simulink model "PatientSimulator_MIMO_toTrim"  (R2022a)
settings: Solver=VariableStepAuto  StartTime=0.0  StopTime=10.0  RelTol=1e-3
undefined symbols (not defined in the file or in its folder): patient, propofol, RASS, remifentanil
libraries: cstblocks x2
settings Model: Creator=user  LastModifiedBy=user

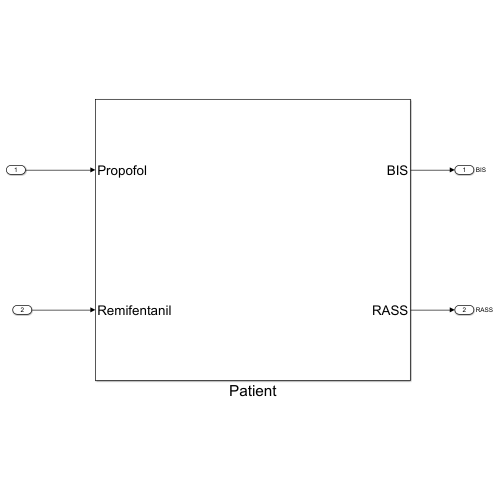
[thumbnail: Simulink's stored preview of the top-level diagram]
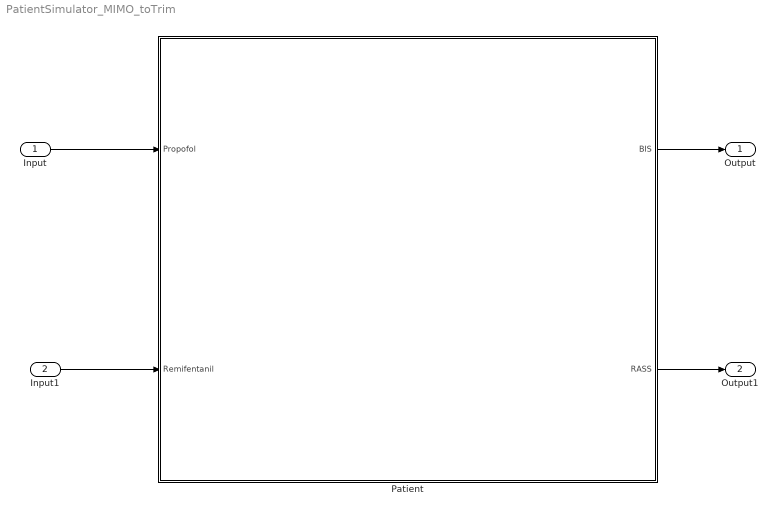
== system PatientSimulator_MIMO_toTrim ==
  Input : Inport
  Input1 : Inport  Port=2
  Patient : Subsystem
  Output : Outport  SignalName=BIS
  Output1 : Outport  Port=2  SignalName=RASS
  wires:
  Input/1 -> Patient/1(Propofol)
  Input1/1 -> Patient/2(Remifentanil)
  Patient/1(BIS) -> Output/1
  Patient/2(RASS) -> Output1/1

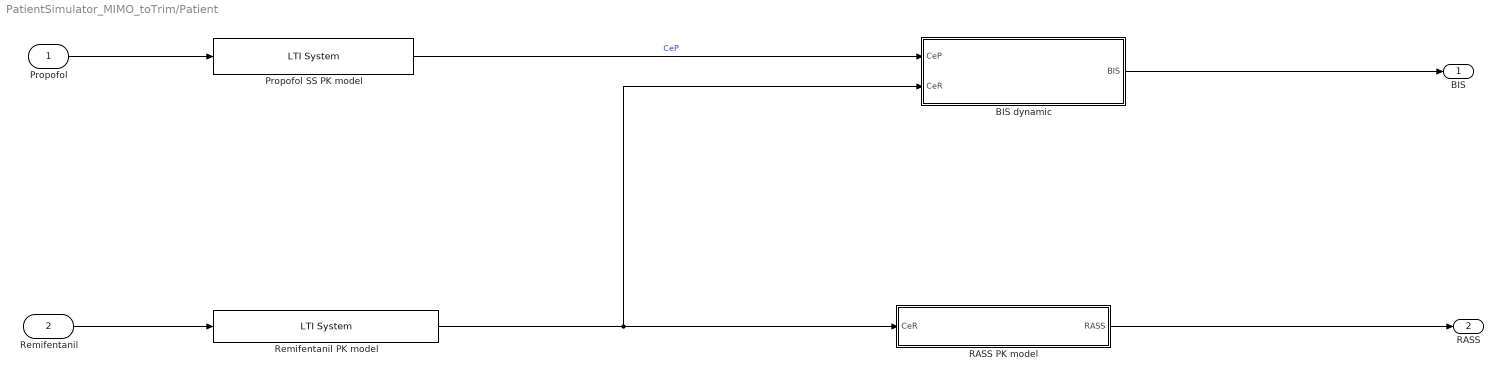
== system PatientSimulator_MIMO_toTrim/Patient ==
  Propofol : Inport
  Remifentanil : Inport  Port=2
  BIS dynamic : Subsystem
  Propofol SS PK model : cstblocks/LTI System  sys=propofol.propSS  IC=0
  RASS PK model : Subsystem
  Remifentanil PK model : cstblocks/LTI System  sys=remifentanil.remiSS  IC=0
  BIS : Outport
  RASS : Outport  Port=2
  wires:
  Propofol SS PK model/1 -> BIS dynamic/1(CeP)  "CeP"
  BIS dynamic/1(BIS) -> BIS/1
  Propofol/1 -> Propofol SS PK model/1
  Remifentanil/1 -> Remifentanil PK model/1
  Remifentanil PK model/1 -> RASS PK model/1(CeR), BIS dynamic/2(CeR)
  RASS PK model/1(RASS) -> RASS/1

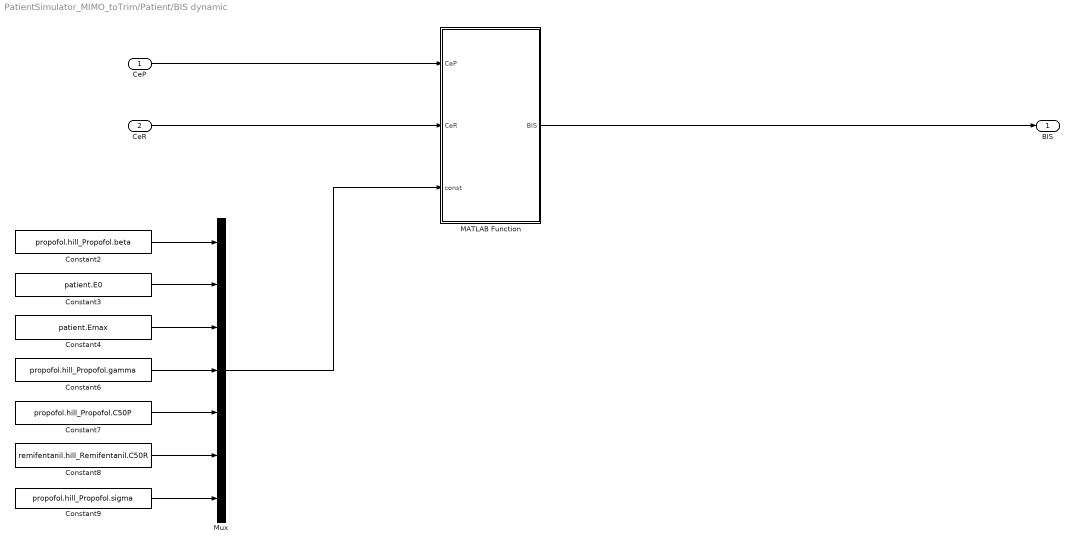
== system PatientSimulator_MIMO_toTrim/Patient/BIS dynamic ==
  CeP : Inport
  CeR : Inport  Port=2
  Constant2 : Constant  Value=propofol.hill_Propofol.beta
  Constant3 : Constant  Value=patient.E0
  Constant4 : Constant  Value=patient.Emax
  Constant6 : Constant  Value=propofol.hill_Propofol.gamma
  Constant7 : Constant  Value=propofol.hill_Propofol.C50P
  Constant8 : Constant  Value=remifentanil.hill_Remifentanil.C50R
  Constant9 : Constant  Value=propofol.hill_Propofol.sigma
  MATLAB Function : MATLAB Function  TreatAsAtomicUnit=on
  Mux : Mux  Inputs=7
  BIS : Outport
  wires:
  Constant9/1 -> Mux/7
  Constant8/1 -> Mux/6
  Constant4/1 -> Mux/3
  Mux/1 -> MATLAB Function/3(const)
  Constant7/1 -> Mux/5
  Constant3/1 -> Mux/2
  Constant6/1 -> Mux/4
  Constant2/1 -> Mux/1
  MATLAB Function/1(BIS) -> BIS/1
  CeP/1 -> MATLAB Function/1(CeP)
  CeR/1 -> MATLAB Function/2(CeR)

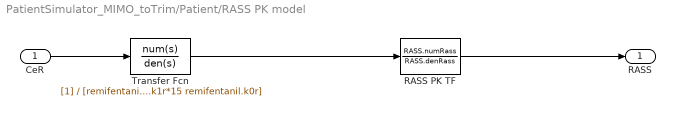
== system PatientSimulator_MIMO_toTrim/Patient/RASS PK model ==
  CeR : Inport
  RASS PK TF : TransferFcn  Numerator=RASS.numRass  Denominator=RASS.denRass
  Transfer Fcn : TransferFcn  Denominator=[remifentanil.k1r*15 remifentanil.k0r]
  RASS : Outport
  wires:
  CeR/1 -> Transfer Fcn/1
  Transfer Fcn/1 -> RASS PK TF/1
  RASS PK TF/1 -> RASS/1

== matlab function PatientSimulator_MIMO_toTrim/Patient/BIS dynamic/MATLAB Function ==
  data: CeP input; BIS output; CeR input; const input
function BIS = fcn(CeP,CeR, const)

if CeP >=0 && CeR >=0
    %% Constant declaration
    beta = const(1);
    E0 = const(2); %starting effect
%     E0 = const(2)-100; %starting effect
    Emax = const(3); %maximum effect achievable
    gamma = const(4); %sigmoidicity
    C50P = const(5); % half effect concentration
    C50R = const(6); % half effect concentration
    sigma = const(7);% sinergy between prop & rem
    
    %% 2D Calculations
    Uprop=CeP./C50P; Uremi=CeR./C50R;
    BIS=E0 - Emax*((Uprop)+(Uremi)+sigma*(Uprop)*(Uremi))^(gamma)/...
        (1+(Uprop+Uremi+sigma*Uprop*Uremi)^(gamma));

else
    BIS = 100;
end
